simulink model "questao2b"  (Simulink 7.1)
settings: Solver=ode45  StartTime=0.0  StopTime=10.0  RelTol=1e-3
settings Model: Creator=ALUNO  LastModifiedBy=ALUNO

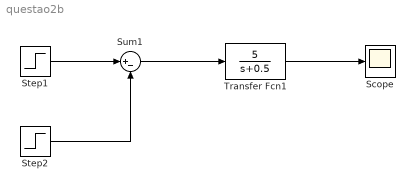
== system questao2b ==
  Scope : Scope
  Step1 : Step  Time=0  After=1/(10*0.2/10)  SampleTime=0
  Step2 : Step  Time=10*0.2/10  After=1/(10*0.2/10)  SampleTime=0
  Sum1 : Sum  Inputs=|+-  OutDataType=sfix(16)  OutScaling=2^0
  Transfer Fcn1 : TransferFcn  Numerator=[5]  Denominator=[1 0.5]
  wires:
  Step1/1 -> Sum1/1
  Step2/1 -> Sum1/2
  Transfer Fcn1/1 -> Scope/1
  Sum1/1 -> Transfer Fcn1/1
